simulink model "EEG_Acquire_SSVEP"  (R2015b)
settings: Solver=FixedStepDiscrete  StartTime=0.0  StopTime=6000  FixedStep=1/250  MaxStep=1/250  RelTol=1e-3
InitFcn:
  | clear global handle
  | 
  | clear global userData
undefined symbols (not defined in the file or in its folder): gcf
libraries: simulink x1
settings Model: Creator=ankit  LastModifiedBy=Nate
settings SolverCC: AutoInsertRateTranBlk=on  InsertRTBMode=Always
settings DataIOCC: LimitDataPoints=off  SaveFormat=Array  SignalLoggingSaveFormat=ModelDataLogs
settings OptimizationCC: ExpressionDepthLimit=2147483647  InitFltsAndDblsToZero=on
settings DebuggingCC: SaveWithParameterizedLinksMsg=none  UnderspecifiedInitializationDetection=Classic  MergeDetectMultiDrivingBlocksExec=none  SignalResolutionControl=TryResolveAllWithWarning  SolverPrmCheckMsg=warning  MultiTaskDSMMsg=warning  MultiTaskCondExecSysMsg=none  FcnCallInpInsideContextMsg=UseLocalSettings  StateNameClashWarn=warning
settings HardwareCC: ProdBitPerPointer=32  ProdLargestAtomicFloat=None  ProdIntDivRoundTo=Undefined  ProdEndianess=Unspecified  ProdWordSize=32  ProdHWDeviceType=32-bit Generic
settings GRTTargetCC: TargetFcnLib=ansi_tfl_tmw.mat  GeneratePreprocessorConditionals=Disable all  CombineOutputUpdateFcns=off  GRTInterface=on
settings ConfigComp: CovModelRefEnable=Off  CovSFcnEnable=off

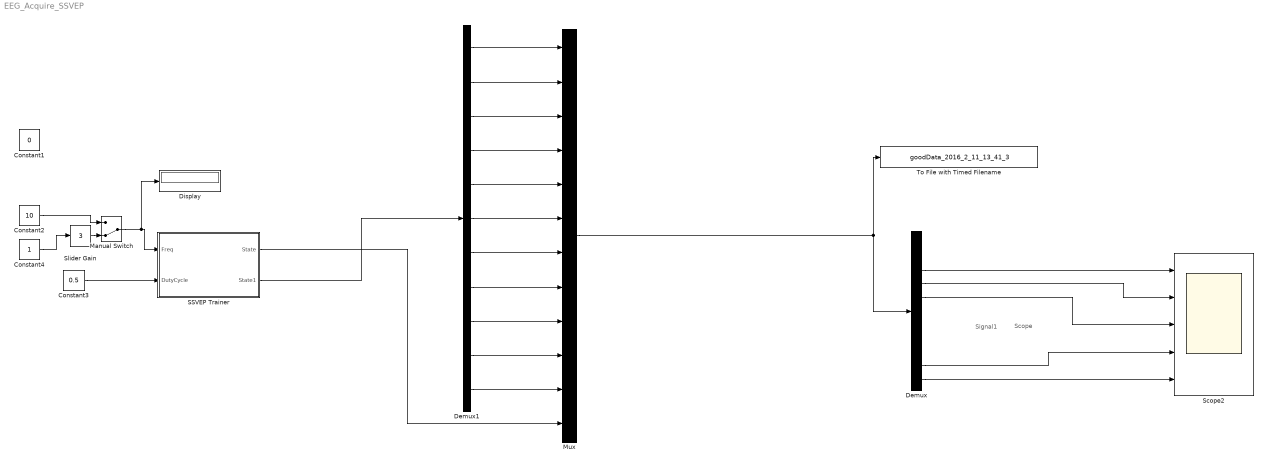
== system EEG_Acquire_SSVEP ==
  note: Scope
  note: Signal1
  Constant1 : Constant  Value=0
  Constant2 : Constant  Value=10
  Constant3 : Constant  Value=0.5
  Constant4 : Constant
  Demux : Demux  Outputs=11
  Demux1 : Demux  Outputs=11
  Display : Display
  Manual Switch : ManualSwitch  CurrentSetting=0
  Mux : Mux  Inputs=12
  SSVEP Trainer : Subsystem  StopFcn=close(gcf)  mask(Single Character Flash Speller){COMPort=COM14, SPS=250}
      mask prompts: COMPort "COM Port"
      mask help: Displays a 36 character matrix. Each character is flashing up for a specific time in a random and sequential order. The dark time is the time between the characters.
      mask Help:
      | Displays a 36 character matrix. Each character is flashing up for a specific time in a random and sequential order. The dark time is the time between the characters. If the character is flashing up the ID-Flash is transmitted for the Signal Processing. Flash contains the ID of every character. Target is one if a specific character for the copy spelling mode flashes up. <br><br>
      | 
      | Mode - can be Copy Spelling or Free Spelling<br><br>
      | Flash time [ms] - time that character is shown on screen <br><br>
      | Dark time [ms] - time between the characters
      mask TypeOptions COMPort: COM1 | COM2 | COM3 | COM4 | COM5 | COM6 | COM7 | COM8 | COM9 | COM10 | COM11 | COM12 | COM13 | COM14 | COM15 | COM16 | COM17 | COM18 | COM19 | COM20
      mask TypeOptions SPS: 250 | 500 | 1000 | 2000 | 4000
      mask Display:
      | port_label('output',2,'EEGData')
      | port_label('output',1,'State')
      | port_label('input',1,'Freq')
      | port_label('input',2,'DutyCycle')
  Scope2 : Scope  NumInputPorts=5
  Slider Gain : simulink/Math Operations/Slider Gain  low=0.5  gain=3  high=100
  To File with Timed Filename : ToFile  InitFcn=|  StopFcn=|  Filename=goodData_2016_2_11_13_41_3  MatrixName=y
      InitFcn=|
      | time=clock;                                                                                                                                                        
      | filenameToFilebase =  get_param(gcb,'Filename');                                                                                                                   
      | rename = [filenameToFilebase '_' num2str(time(1)) '_' num2str(time(2)) '_' num2str(time(3)) '_' num2str(time(4)) '_' num2str(time(5)) '_' num2str(round(time(6)))];
      | set_param(gcb,'Filename',rename);                                 clear time;                                                       clear rename;
      StopFcn=|
      | set_param(gcb,'Filename',filenameToFilebase);
      |                                              
      | clear filenameToFilebase
      settings: AttributesFormatString=Enter Base name, time will be added
  wires:
  Demux/5 -> Scope2/3
  Demux/3 -> Scope2/1
  Demux/4 -> Scope2/2
  Demux/11 -> Scope2/5
  Demux/10 -> Scope2/4
  Demux1/4 -> Mux/4
  Demux1/2 -> Mux/2
  Demux1/1 -> Mux/1
  Demux1/9 -> Mux/9
  Demux1/8 -> Mux/8
  Demux1/7 -> Mux/7
  Demux1/6 -> Mux/6
  Demux1/11 -> Mux/11
  Demux1/10 -> Mux/10
  Demux1/3 -> Mux/3
  Demux1/5 -> Mux/5
  SSVEP Trainer/2(State1) -> Demux1/1
  SSVEP Trainer/1(State) -> Mux/12
  Constant3/1 -> SSVEP Trainer/2(DutyCycle)
  Constant2/1 -> Manual Switch/1
  Manual Switch/1 -> Display/1, SSVEP Trainer/1(Freq)
  Mux/1 -> Demux/1, To File with Timed Filename/1
  Constant4/1 -> Slider Gain/1
  Slider Gain/1 -> Manual Switch/2

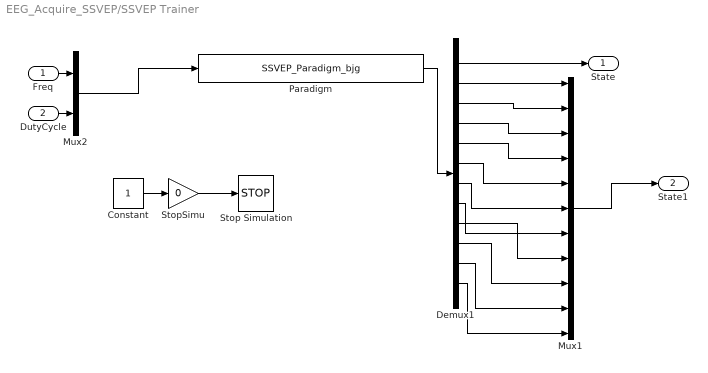
== system EEG_Acquire_SSVEP/SSVEP Trainer ==
  Freq : Inport
  DutyCycle : Inport  Port=2
  Constant : Constant
  Demux1 : Demux  Outputs=12
  Mux1 : Mux  Inputs=11
  Mux2 : Mux  Inputs=2
  Paradigm : S-Function  FunctionName=SSVEP_Paradigm_bjg  Parameters=COMPort,SPS  SFunctionDeploymentMode=off  EnableBusSupport=off
  Stop Simulation : Stop
  StopSimu : Gain  Gain=0
  State : Outport
  State1 : Outport  Port=2
  wires:
  Paradigm/1 -> Demux1/1
  Constant/1 -> StopSimu/1
  StopSimu/1 -> Stop Simulation/1
  Mux1/1 -> State1/1
  Mux2/1 -> Paradigm/1
  Demux1/2 -> Mux1/1
  Demux1/3 -> Mux1/2
  Demux1/4 -> Mux1/3
  Demux1/5 -> Mux1/4
  Demux1/6 -> Mux1/5
  Demux1/7 -> Mux1/6
  Demux1/8 -> Mux1/7
  Demux1/9 -> Mux1/8
  Demux1/10 -> Mux1/9
  Demux1/11 -> Mux1/10
  Demux1/12 -> Mux1/11
  Demux1/1 -> State/1
  Freq/1 -> Mux2/1
  DutyCycle/1 -> Mux2/2
